simulink library "offsetLeadDistance_ul"  (R2018a)
settings: Solver=VariableStepAuto  StartTime=0.0  StopTime=10.0  RelTol=1e-3
values from neighbouring files (symbols this model uses):
  offsetLeadDistance_none = 0.02    [offsetLeadDistance_init.m]
settings Model: Creator=mcobb  LastModifiedBy=mcobb

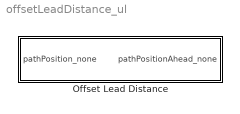
== system offsetLeadDistance_ul ==
  Offset Lead Distance : Subsystem

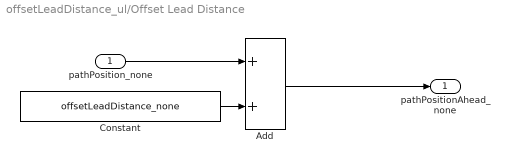
== system offsetLeadDistance_ul/Offset Lead Distance ==
  pathPosition_none : Inport
  Add : Sum
  Constant : Constant  Value=offsetLeadDistance_none
  pathPositionAhead_none : Outport
  wires:
  pathPosition_none/1 -> Add/1
  Add/1 -> pathPositionAhead_none/1
  Constant/1 -> Add/2
